simulink model "Mocap"  (R2017b)
settings: Solver=VariableStepAuto  StartTime=0.0  StopTime=100  RelTol=1e-3
libraries: instrumentlib x1, slrtlib x1, xpcrtudplib x1, dspnetwork x1
settings Model: Creator=RoahmLab  LastModifiedBy=RoahmLab

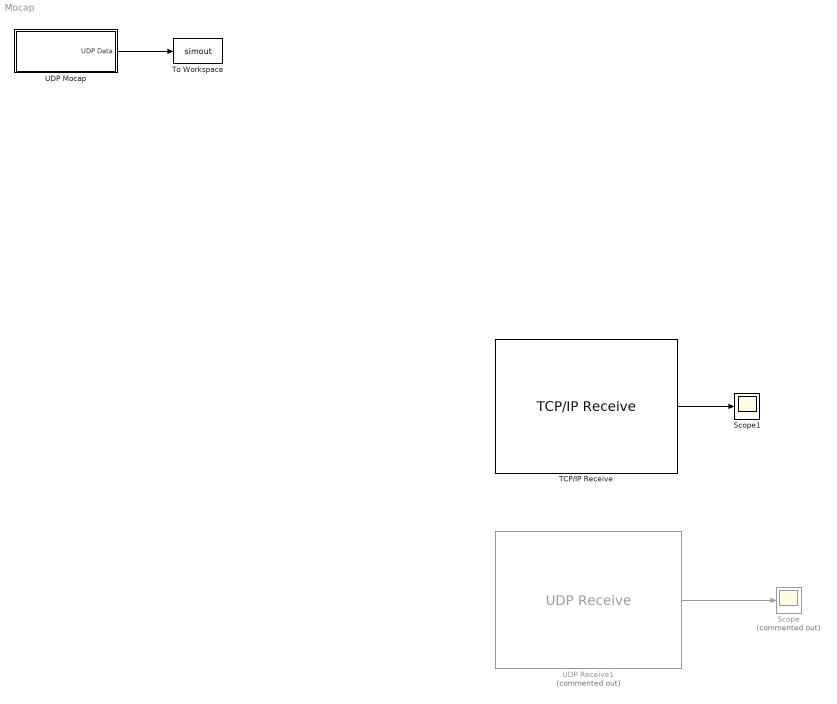
== system Mocap ==
  Scope : Scope  Commented=on
  Scope1 : Scope
  TCP/IP Receive : instrumentlib/TCP//IP Receive  Host=127.0.0.1  Port=11000  DataSize="[3  3]"  EnableBlockingMode=on  Timeout=10  SampleTime=0.01  DataType=double  ByteOrder=LittleEndian
      settings: SourceProductName=Instrument Control Toolbox
  To Workspace : ToWorkspace  VariableName=simout  SaveFormat=Timeseries  SampleTime=-1
  "UDP Mocap " : Subsystem
  UDP Receive1 : dspnetwork/UDP Receive  Commented=on  localURL='0.0.0.0'  localPort=11000  remoteURL='192.168.1.23'  remotePort=-1  recvBufferSize=24  dims=255  signalDatatype=double  isVarSize=on  showBlockingTime=off  blockingTime=0  sampletime=1  blockPlatform=[]
      settings: SourceProductName=DSP System Toolbox  SourceProductBaseCode=DS
  wires:
  "UDP Mocap "/1(UDP Data) -> To Workspace/1
  UDP Receive1/1 -> Scope/1
  TCP/IP Receive/1 -> Scope1/1

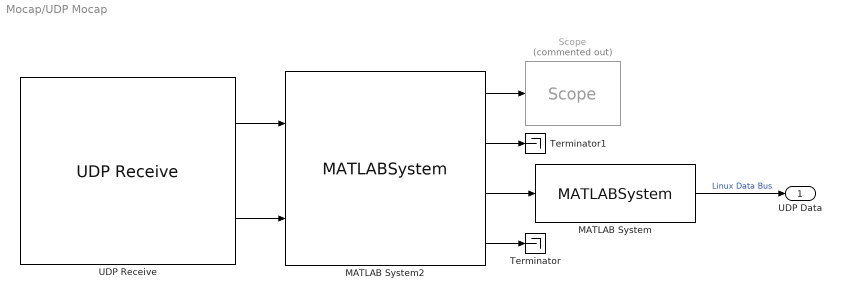
== system Mocap/UDP Mocap  ==
  MATLAB System : MATLABSystem  System=BytesToCassieMocapDataBus  SimulateUsing=Interpreted execution
      mask Type: BytesToCassieMocapDataBus
      mask Display: disp('BytesToCassieMocapDataBus');
  MATLAB System2 : MATLABSystem  System=ProcessUdpMocapPacket  heartbeatInterval=0.01  HeaderLength=0  CassieLinuxDataLength=24  SimulateUsing=Interpreted execution
      mask Type: ProcessUdpMocapPacket
      mask Display:
      | disp('ProcessUdpMocapPacket');
      | port_label('input',1,'UDP Data');
      | port_label('input',2,'Length');
      | port_label('output',1,'Log');
      | port_label('output',2,'Header');
      | port_label('output',3,'LinuxData');
      | port_label('output',4,'timeout');
  "Scope " : slrtlib/Displays and Logging/Scope   Commented=on  scopeno=1  scopetype=File  autostart=on  viewmode=Graphical redraw  formatstr='%15.6f'  grid=on  ylimits=[0,0]  nosamples=250  noprepostsamples=0  interleave=1  triggermode=FreeRun  triggersignal=1  trigsignalfromport=off  triggerlevel=0.0  triggerslope=Either  triggerscope=1  triggersample=0  filename=udp.dat  mode=Commit  writesize=4096  autorestart=on  dynamicfilemode=off  maxwritefilesize=2048*1024^2 - 4096
  Terminator : Terminator
  Terminator1 : Terminator
  UDP Receive : xpcrtudplib/UDP Receive  ipAddressVal=Use host-target connection  localPort=11000  rcvWidth=24  rcvFmAny=off  fmAddress=127.0.0.1  maxUDPQueue=8  sampleTime=-1
      settings: SourceProductName=Simulink Real-Time
  UDP Data : Outport
  wires:
  MATLAB System2/3 -> MATLAB System/1
  MATLAB System2/1 -> "Scope "/1
  UDP Receive/2 -> MATLAB System2/2
  UDP Receive/1 -> MATLAB System2/1
  MATLAB System/1 -> UDP Data/1  "Linux Data Bus"
  MATLAB System2/4 -> Terminator/1
  MATLAB System2/2 -> Terminator1/1
